simulink library "lib_Clutchless_HSC"  (R2017b)
settings: Solver=VariableStepAuto  StartTime=0.0  StopTime=10.0  RelTol=1e-3
undefined symbols (not defined in the file): cal, eng, Engine, ENGTRQ_MSMCH_Degraded_CP, ENGTRQ_MSMCH_ErrCritical_CP, ENGTRQ_MSMCH_LimpHome_CP, gb, mot, tloop
libraries: simulink x83, EC2_libraries x4, powerlib_meascontrol x2, lib_SystemDiag x1, dspsigops x1
(part 4 of 6)

== system lib_Clutchless_HSC/Clutchless_HSC/HSC/Powertrain Manager/Torque Distribution/Supervisory  Control  Logic/VehReady.Sport_Mode.EngTrqCalc ==
  APP : Inport
  EngSpeed : Inport  Port=2
  Shifter : Inport  Port=3
  DrvIntdAxleTrq : Inport  Port=4
  TransRatio : Inport  Port=5
  f : TriggerPort  TriggerType=function-call  VariantControl=Variant
      settings: CopyFcn=Stateflow.SLINSF.SimulinkMan.removeBlockPreDeleteFcn  PreDeleteFcn=Stateflow.SLINSF.SimulinkMan.unsafePredeleteFcn
  Constant : Constant  Value=0
  Constant1 : Constant  Value=0
  Divide2 : Product  Inputs=**
  Divide3 : Product  Inputs=***
  Engine Max Trq : Lookup_n-D  NumberOfTableDimensions=1  BreakpointsForDimension1="[600\t800\t1000\t1200\t1400\t1600\t1800\t2000\t2200\t2400\t2600\t2800\t3000\t3200\t3400\t3600\t3800\t4000\t4250\t4500\t4750\t5000\t5250\t5500\t5750\t6000\t6250\t6500]"  Table="[83.7900000000000\t136.760000000000\t140\t152.010000000000\t171.590000000000\t185.900000000000\t198.400000000000\t197.360000000000\t200.550000000000\t202.260000000000\t215.080000000000\t204.810000000000\t204.520000000000\t208.100000000000\t211.520000000000\t210.560000000000\t214.100000000000\t213.470000000000\t208.730000000000\t208.430000000000\t208.670000000000\t231.210000000000\t228.310000000000\t225.330000000000\t220.520000000000\t211.210000000000\t204.190000000000\t151.770000000000]"  ExtrapMethod=Clip  UseLastTableValue=on  InternalRulePriority=Speed  RndMeth=Simplest  InputSameDT=on
  Final Drive Ratio : Constant  Value=fd.plant.init.ratio
  Index Vector : MultiPortSwitch  DataPortOrder=Zero-based contiguous  Inputs=5  zeroidx=on
  MinMax : MinMax  Inputs=2
  Saturation : Saturate  UpperLimit=230  LowerLimit=-inf
  to% : Gain  Gain=1/100
  T : Outport
  wires:
  MinMax/1 -> [TrqCalc]
  DrvIntdAxleTrq/1 -> MinMax/2
  Divide3/1 -> MinMax/1
  Final Drive Ratio/1 -> Divide3/3
  TransRatio/1 -> Divide3/2
  Divide2/1 -> Divide3/1
  Saturation/1 -> Divide2/2
  Engine Max Trq/1 -> Saturation/1
  EngSpeed/1 -> Engine Max Trq/1  "RPM"
  to%/1 -> Divide2/1
  APP/1 -> to%/1
  Shifter/1 -> Index Vector/1
  Index Vector/1 -> T/1
  [TrqCalc] -> Index Vector/5  "N"
  Constant1/1 -> Index Vector/3  "P"
  Constant/1 -> Index Vector/2  "Between Ranges"
  [TrqCalc] -> Index Vector/6  "D"
  [TrqCalc] -> Index Vector/4  "R"

== system lib_Clutchless_HSC/Clutchless_HSC/HSC/Powertrain Manager/Torque Distribution/Supervisory  Control  Logic/VehReady.Sport_Mode.MotTrqCalc ==
  APP : Inport
  Shifter : Inport  Port=2
  MotSpeed : Inport  Port=3
  DrvIntdAxleTrq : Inport  Port=4
  TransRatio : Inport  Port=5
  f : TriggerPort  TriggerType=function-call  VariantControl=Variant
      settings: CopyFcn=Stateflow.SLINSF.SimulinkMan.removeBlockPreDeleteFcn  PreDeleteFcn=Stateflow.SLINSF.SimulinkMan.unsafePredeleteFcn
  % to 1 : Gain  Gain=1/100
  Constant : Constant  Value=0
  Constant1 : Constant  Value=0
  Differential Ratio : Constant  Value=fd.plant.init.ratio
  Divide1 : Product  Inputs=**
  Divide2 : Product  Inputs=***
  Index Vector : MultiPortSwitch  DataPortOrder=Zero-based contiguous  Inputs=5  zeroidx=on
  MinMax : MinMax  Inputs=2
  Peak trq max - Motoring : Lookup  InputValues=mot.plant.init.regen.trq_max.idx1_spd  Table=mot.plant.init.motor.trq_max.map  LookUpMeth=Interpolation-Use End Values  SaturateOnIntegerOverflow=on
  T : Outport
  wires:
  MinMax/1 -> [TrqCalc]
  Divide2/1 -> MinMax/2
  DrvIntdAxleTrq/1 -> MinMax/1
  Differential Ratio/1 -> Divide2/3
  TransRatio/1 -> Divide2/2
  Divide1/1 -> Divide2/1
  Peak trq max - Motoring/1 -> Divide1/1
  MotSpeed/1 -> Peak trq max - Motoring/1  "RPM"
  APP/1 -> % to 1/1
  [TrqCalc] -> Index Vector/5  "N"
  Constant1/1 -> Index Vector/3  "P"
  Constant/1 -> Index Vector/2  "Between Ranges"
  Index Vector/1 -> T/1
  [TrqCalc] -> Index Vector/6  "D"
  [TrqCalc] -> Index Vector/4  "R"
  Shifter/1 -> Index Vector/1
  % to 1/1 -> Divide1/2

== system lib_Clutchless_HSC/Clutchless_HSC/HSC/Powertrain Manager/Torque Distribution/SysPwrMd ==
  note: Disable Engine if HVIL on
  note: Switch added to test engine start
      | 04/13/2017 - Sebastian
  SysPwrMd : Inport
  EngRunAtv : Inport  Port=2
  EngOnReq : Inport  Port=3
  Fehler_Pilot : Inport  Port=4
  Constant1 : Constant  Value=3
  Constant2 : Constant
  Constant3 : Constant  Value=0
  EngOnReq_Cal : Constant  Value=0
  Saturation2 : Saturate  UpperLimit=2  LowerLimit=0
  Saturation3 : Saturate  UpperLimit=2  LowerLimit=0
  Switch{1..5} (5 alike) : Switch  Threshold=1
  Out1 : Outport
  wires:
  Switch2/1 -> Switch3/3
  Constant1/1 -> Switch1/3
  Constant2/1 -> Switch2/1
  EngRunAtv/1 -> Switch2/2, Switch1/2
  Saturation2/1 -> Switch1/1
  SysPwrMd/1 -> Saturation3/1, Saturation2/1
  Saturation3/1 -> Switch2/3
  EngOnReq/1 -> Switch4/3
  Switch1/1 -> Switch3/1
  Switch3/1 -> Switch5/3
  EngOnReq_Cal/1 -> Switch4/2, Switch4/1
  Switch4/1 -> Switch3/2
  Fehler_Pilot/1 -> Switch5/2
  Switch5/1 -> Out1/1
  Constant3/1 -> Switch5/1

== system lib_Clutchless_HSC/Clutchless_HSC/HSC/Powertrain Manager/Torque Distribution/eSystemStatusValidity ==
  In1 : Inport
  " Normal Operation" : simulink/Logic and Bit Operations/Compare To Constant  relop===  const=2  OutDataTypeStr=boolean
  Limited Operation : simulink/Logic and Bit Operations/Compare To Constant  relop===  const=1  OutDataTypeStr=boolean
  Logical Operator : Logic  Operator=OR  AllPortsSameDT=off  OutDataTypeStr=boolean
  Out1 : Outport
  wires:
  In1/1 -> " Normal Operation"/1, Limited Operation/1
  Limited Operation/1 -> Logical Operator/1
  " Normal Operation"/1 -> Logical Operator/2
  Logical Operator/1 -> Out1/1

== system lib_Clutchless_HSC/Clutchless_HSC/HSC/Powertrain Manager/Torque Distribution/iceSystemStatusValidity ==
  In1 : Inport
  " Normal Operation" : simulink/Logic and Bit Operations/Compare To Constant  relop===  const=2  OutDataTypeStr=boolean
  Limited Operation : simulink/Logic and Bit Operations/Compare To Constant  relop===  const=1  OutDataTypeStr=boolean
  Logical Operator : Logic  Operator=OR  AllPortsSameDT=off  OutDataTypeStr=boolean
  Out1 : Outport
  wires:
  Logical Operator/1 -> Out1/1
  " Normal Operation"/1 -> Logical Operator/2
  Limited Operation/1 -> Logical Operator/1
  In1/1 -> Limited Operation/1, " Normal Operation"/1

== system lib_Clutchless_HSC/Clutchless_HSC/HSC/Camaro Fault Detection/Component Diagnostic/Engine Component Diagnostic/Override  engTrqCmd ==
  note: Override Switch Subsystem
  note: This subsystem is used to override the model value of a signal to a constant value
  In1 : Inport
  Constant : Constant  Value=50
  Multiport Switch : MultiPortSwitch  DataPortOrder=Zero-based contiguous  Inputs=2  zeroidx=on
  Signal Override Switch 0 = Use Model 1 = Use Constant : Constant
  Out1 : Outport
  wires:
  Constant/1 -> Multiport Switch/3
  Multiport Switch/1 -> Out1/1
  In1/1 -> Multiport Switch/2
  Signal Override Switch 0 = Use Model 1 = Use Constant/1 -> Multiport Switch/1

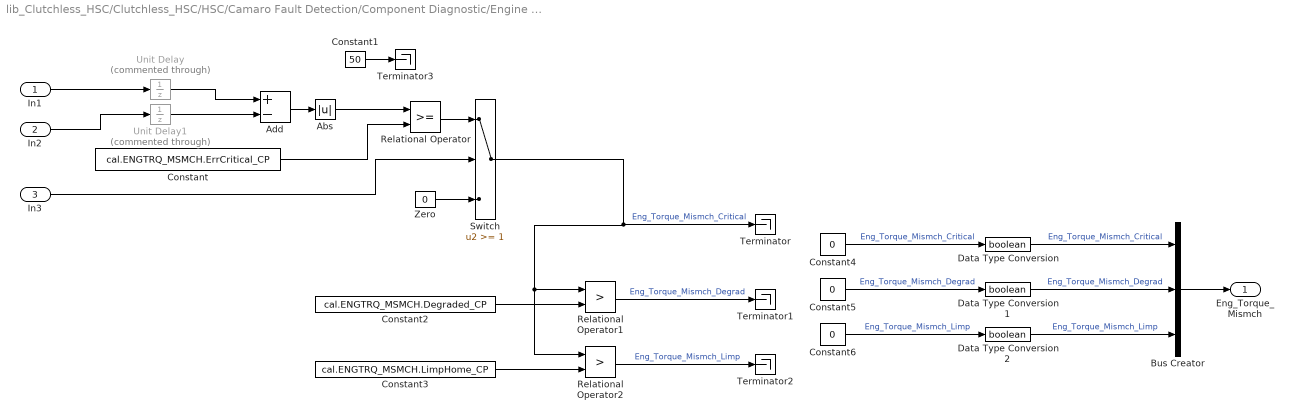
== system lib_Clutchless_HSC/Clutchless_HSC/HSC/Camaro Fault Detection/Component Diagnostic/Engine Component Diagnostic/TorqMismatch Detection ==
  In1 : Inport
  In2 : Inport  Port=2
  In3 : Inport  Port=3
  Abs : Abs
  Add : Sum  Inputs=+-
  Bus Creator : BusCreator  Inputs=3
  Constant : Constant  Value=cal.ENGTRQ_MSMCH.ErrCritical_CP
  Constant1 : Constant  Value=50
  Constant2 : Constant  Value=cal.ENGTRQ_MSMCH.Degraded_CP
  Constant3 : Constant  Value=cal.ENGTRQ_MSMCH.LimpHome_CP
  Constant4 : Constant  Value=0
  Constant5 : Constant  Value=0
  Constant6 : Constant  Value=0
  Data Type Conversion : DataTypeConversion  OutDataTypeStr=boolean
  Data Type Conversion1 : DataTypeConversion  OutDataTypeStr=boolean
  Data Type Conversion2 : DataTypeConversion  OutDataTypeStr=boolean
  Relational Operator : RelationalOperator  OutDataTypeStr=boolean  RndMeth=Nearest
  Relational Operator1 : RelationalOperator  Operator=>  OutDataTypeStr=boolean  RndMeth=Nearest
  Relational Operator2 : RelationalOperator  Operator=>  OutDataTypeStr=boolean  RndMeth=Nearest
  Switch : Switch  Threshold=1
  Terminator{,1..3} (4 alike) : Terminator
  Unit Delay : UnitDelay  Commented=through  SampleTime=-1
  Unit Delay1 : UnitDelay  Commented=through  SampleTime=-1
  "Zero " : Constant  Value=0
  Eng_Torque_Mismch : Outport
  wires:
  Data Type Conversion2/1 -> Bus Creator/3  "Eng_Torque_Mismch_Limp"
  Data Type Conversion1/1 -> Bus Creator/2  "Eng_Torque_Mismch_Degrad"
  Data Type Conversion/1 -> Bus Creator/1  "Eng_Torque_Mismch_Critical"
  Constant5/1 -> Data Type Conversion1/1  "Eng_Torque_Mismch_Degrad"
  Constant6/1 -> Data Type Conversion2/1  "Eng_Torque_Mismch_Limp"
  Constant4/1 -> Data Type Conversion/1  "Eng_Torque_Mismch_Critical"
  Abs/1 -> Relational Operator/1
  Unit Delay1/1 -> Add/2
  Bus Creator/1 -> Eng_Torque_Mismch/1
  Relational Operator2/1 -> Terminator2/1  "Eng_Torque_Mismch_Limp"
  Relational Operator1/1 -> Terminator1/1  "Eng_Torque_Mismch_Degrad"
  Constant3/1 -> Relational Operator2/2
  Constant2/1 -> Relational Operator1/2
  Switch/1 -> Terminator/1, Relational Operator1/1, Relational Operator2/1  "Eng_Torque_Mismch_Critical"
  Relational Operator/1 -> Switch/1
  Add/1 -> Abs/1
  Constant/1 -> Relational Operator/2
  Unit Delay/1 -> Add/1
  In3/1 -> Switch/2
  "Zero "/1 -> Switch/3
  In2/1 -> Unit Delay1/1
  In1/1 -> Unit Delay/1
  Constant1/1 -> Terminator3/1

== system lib_Clutchless_HSC/Clutchless_HSC/HSC/Camaro Fault Detection/Input Conversions/BMS_Conversions/Override  BMS_gdf 0_1 ==
  note: This subsystem is used to override the model value of a signal to a constant value
  note: Override Switch Subsystem
  In1 : Inport
  Multiport Switch : MultiPortSwitch  DataPortOrder=Zero-based contiguous  Inputs=2  zeroidx=on
  Override Value : Constant  Value=0  OutDataTypeStr=double
  Signal Override Switch 0 = Use Model 1 = Use Constant : Constant
  Out1 : Outport
  wires:
  Signal Override Switch 0 = Use Model 1 = Use Constant/1 -> Multiport Switch/1
  In1/1 -> Multiport Switch/2
  Multiport Switch/1 -> Out1/1
  Override Value/1 -> Multiport Switch/3

== system lib_Clutchless_HSC/Clutchless_HSC/HSC/Camaro Fault Detection/Input Conversions/BMS_Conversions/Override  closeContactorsCmd ==
  note: Override Switch Subsystem
  note: This subsystem is used to override the model value of a signal to a constant value
  In1 : Inport
  Multiport Switch : MultiPortSwitch  DataPortOrder=Zero-based contiguous  Inputs=2  zeroidx=on
  Override Value : Constant  Value=0  OutDataTypeStr=double
  Signal Override Switch 0 = Use Model 1 = Use Constant : Constant  Value=0
  Out1 : Outport
  wires:
  Override Value/1 -> Multiport Switch/3
  Multiport Switch/1 -> Out1/1
  In1/1 -> Multiport Switch/2
  Signal Override Switch 0 = Use Model 1 = Use Constant/1 -> Multiport Switch/1

== system lib_Clutchless_HSC/Clutchless_HSC/HSC/Camaro Fault Detection/Input Conversions/BMS_Conversions/Override  contactorsClsd ==
  note: Override Switch Subsystem
  note: This subsystem is used to override the model value of a signal to a constant value
  In1 : Inport
  Multiport Switch : MultiPortSwitch  DataPortOrder=Zero-based contiguous  Inputs=2  zeroidx=on
  Override Value : Constant  Value=0  OutDataTypeStr=double
  Signal Override Switch 0 = Use Model 1 = Use Constant : Constant  Value=0
  Out1 : Outport
  wires:
  Override Value/1 -> Multiport Switch/3
  Multiport Switch/1 -> Out1/1
  In1/1 -> Multiport Switch/2
  Signal Override Switch 0 = Use Model 1 = Use Constant/1 -> Multiport Switch/1

== system lib_Clutchless_HSC/Clutchless_HSC/HSC/Camaro Fault Detection/Input Conversions/BMS_Conversions/Override  essCur_A ==
  note: This subsystem is used to override the model value of a signal to a constant value
  note: Override Switch Subsystem
  In1 : Inport
  Multiport Switch : MultiPortSwitch  DataPortOrder=Zero-based contiguous  Inputs=2  zeroidx=on
  Override Value : Constant  Value=0  OutDataTypeStr=double
  Signal Override Switch 0 = Use Model 1 = Use Constant : Constant  Value=0
  Out1 : Outport
  wires:
  Signal Override Switch 0 = Use Model 1 = Use Constant/1 -> Multiport Switch/1
  In1/1 -> Multiport Switch/2
  Multiport Switch/1 -> Out1/1
  Override Value/1 -> Multiport Switch/3

== system lib_Clutchless_HSC/Clutchless_HSC/HSC/Camaro Fault Detection/Input Conversions/BMS_Conversions/Override  essSOC_0_1 ==
  note: Override Switch Subsystem
  note: This subsystem is used to override the model value of a signal to a constant value
  In1 : Inport
  Multiport Switch : MultiPortSwitch  DataPortOrder=Zero-based contiguous  Inputs=2  zeroidx=on
  Override Value : Constant  Value=0  OutDataTypeStr=double
  Signal Override Switch 0 = Use Model 1 = Use Constant : Constant  Value=0
  Out1 : Outport
  wires:
  Override Value/1 -> Multiport Switch/3
  Multiport Switch/1 -> Out1/1
  In1/1 -> Multiport Switch/2
  Signal Override Switch 0 = Use Model 1 = Use Constant/1 -> Multiport Switch/1

== system lib_Clutchless_HSC/Clutchless_HSC/HSC/Camaro Fault Detection/Input Conversions/BMS_Conversions/Override  essTemp_C ==
  note: Override Switch Subsystem
  note: This subsystem is used to override the model value of a signal to a constant value
  In1 : Inport
  Multiport Switch : MultiPortSwitch  DataPortOrder=Zero-based contiguous  Inputs=2  zeroidx=on
  Override Value : Constant  Value=0  OutDataTypeStr=double
  Signal Override Switch 0 = Use Model 1 = Use Constant : Constant
  Out1 : Outport
  wires:
  Override Value/1 -> Multiport Switch/3
  Multiport Switch/1 -> Out1/1
  In1/1 -> Multiport Switch/2
  Signal Override Switch 0 = Use Model 1 = Use Constant/1 -> Multiport Switch/1

== system lib_Clutchless_HSC/Clutchless_HSC/HSC/Camaro Fault Detection/Input Conversions/BMS_Conversions/Override  hvBattVolt_V ==
  note: Override Switch Subsystem
  note: This subsystem is used to override the model value of a signal to a constant value
  In1 : Inport
  Multiport Switch : MultiPortSwitch  DataPortOrder=Zero-based contiguous  Inputs=2  zeroidx=on
  Override Value : Constant  Value=0  OutDataTypeStr=double
  Signal Override Switch 0 = Use Model 1 = Use Constant : Constant  Value=0
  Out1 : Outport
  wires:
  Override Value/1 -> Multiport Switch/3
  Multiport Switch/1 -> Out1/1
  In1/1 -> Multiport Switch/2
  Signal Override Switch 0 = Use Model 1 = Use Constant/1 -> Multiport Switch/1

== system lib_Clutchless_HSC/Clutchless_HSC/HSC/Camaro Fault Detection/Input Conversions/BMS_Conversions/Override  hvBusVolt_V ==
  note: This subsystem is used to override the model value of a signal to a constant value
  note: Override Switch Subsystem
  In1 : Inport
  Multiport Switch : MultiPortSwitch  DataPortOrder=Zero-based contiguous  Inputs=2  zeroidx=on
  Override Value : Constant  Value=0  OutDataTypeStr=double
  Signal Override Switch 0 = Use Model 1 = Use Constant : Constant  Value=0
  Out1 : Outport
  wires:
  Signal Override Switch 0 = Use Model 1 = Use Constant/1 -> Multiport Switch/1
  In1/1 -> Multiport Switch/2
  Multiport Switch/1 -> Out1/1
  Override Value/1 -> Multiport Switch/3

== system lib_Clutchless_HSC/Clutchless_HSC/HSC/Camaro Fault Detection/Input Conversions/BMS_Conversions/Override  rollingAliveCnt [1_3] ==
  note: This subsystem is used to override the model value of a signal to a constant value
  note: Override Switch Subsystem
  In1 : Inport
  Multiport Switch : MultiPortSwitch  DataPortOrder=Zero-based contiguous  Inputs=2  zeroidx=on
  Override Value : Constant  Value=0  OutDataTypeStr=double
  Signal Override Switch 0 = Use Model 1 = Use Constant : Constant  Value=0
  Out1 : Outport
  wires:
  Signal Override Switch 0 = Use Model 1 = Use Constant/1 -> Multiport Switch/1
  In1/1 -> Multiport Switch/2
  Multiport Switch/1 -> Out1/1
  Override Value/1 -> Multiport Switch/3

== system lib_Clutchless_HSC/Clutchless_HSC/HSC/Camaro Fault Detection/Input Conversions/BMS_Conversions/Override Fehler_HS_offen ==
  note: Override Switch Subsystem
  note: This subsystem is used to override the model value of a signal to a constant value
  In1 : Inport
  Multiport Switch : MultiPortSwitch  DataPortOrder=Zero-based contiguous  Inputs=2  zeroidx=on
  Override Value : Constant  Value=0  OutDataTypeStr=double
  Signal Override Switch 0 = Use Model 1 = Use Constant : Constant
  Out1 : Outport
  wires:
  Override Value/1 -> Multiport Switch/3
  Multiport Switch/1 -> Out1/1
  In1/1 -> Multiport Switch/2
  Signal Override Switch 0 = Use Model 1 = Use Constant/1 -> Multiport Switch/1

== system lib_Clutchless_HSC/Clutchless_HSC/HSC/Camaro Fault Detection/Input Conversions/BMS_Conversions/Override Fehler_HS_verschweisst ==
  note: This subsystem is used to override the model value of a signal to a constant value
  note: Override Switch Subsystem
  In1 : Inport
  Multiport Switch : MultiPortSwitch  DataPortOrder=Zero-based contiguous  Inputs=2  zeroidx=on
  Override Value : Constant  Value=0  OutDataTypeStr=double
  Signal Override Switch 0 = Use Model 1 = Use Constant : Constant
  Out1 : Outport
  wires:
  Signal Override Switch 0 = Use Model 1 = Use Constant/1 -> Multiport Switch/1
  In1/1 -> Multiport Switch/2
  Multiport Switch/1 -> Out1/1
  Override Value/1 -> Multiport Switch/3

== system lib_Clutchless_HSC/Clutchless_HSC/HSC/Camaro Fault Detection/Input Conversions/DriverInput_Conversions/Override  KeyPos [0_3] ==
  note: This subsystem is used to override the model value of a signal to a constant value
  note: Override Switch Subsystem
  In1 : Inport
  Multiport Switch : MultiPortSwitch  DataPortOrder=Zero-based contiguous  Inputs=2  zeroidx=on
  Override Value : Constant  Value=0  OutDataTypeStr=double
  Signal Override Switch 0 = Use Model 1 = Use Constant : Constant  Value=0
  Out1 : Outport
  wires:
  Signal Override Switch 0 = Use Model 1 = Use Constant/1 -> Multiport Switch/1
  In1/1 -> Multiport Switch/2
  Multiport Switch/1 -> Out1/1
  Override Value/1 -> Multiport Switch/3

== system lib_Clutchless_HSC/Clutchless_HSC/HSC/Camaro Fault Detection/Input Conversions/DriverInput_Conversions/Override APP (%) ==
  note: This subsystem is used to override the model value of a signal to a constant value
  note: Override Switch Subsystem
  In1 : Inport
  Multiport Switch : MultiPortSwitch  DataPortOrder=Zero-based contiguous  Inputs=2  zeroidx=on
  Override Value : Constant  Value=0  OutDataTypeStr=double
  Signal Override Switch 0 = Use Model 1 = Use Constant : Constant  Value=0
  Out1 : Outport
  wires:
  Signal Override Switch 0 = Use Model 1 = Use Constant/1 -> Multiport Switch/1
  In1/1 -> Multiport Switch/2
  Multiport Switch/1 -> Out1/1
  Override Value/1 -> Multiport Switch/3

== system lib_Clutchless_HSC/Clutchless_HSC/HSC/Camaro Fault Detection/Input Conversions/DriverInput_Conversions/Override APP (%)1 ==
  note: Override Switch Subsystem
  note: This subsystem is used to override the model value of a signal to a constant value
  In1 : Inport
  Multiport Switch : MultiPortSwitch  DataPortOrder=Zero-based contiguous  Inputs=2  zeroidx=on
  Override Value : Constant  Value=0  OutDataTypeStr=double
  Signal Override Switch 0 = Use Model 1 = Use Constant : Constant  Value=0
  Out1 : Outport
  wires:
  Override Value/1 -> Multiport Switch/3
  Multiport Switch/1 -> Out1/1
  In1/1 -> Multiport Switch/2
  Signal Override Switch 0 = Use Model 1 = Use Constant/1 -> Multiport Switch/1

== system lib_Clutchless_HSC/Clutchless_HSC/HSC/Camaro Fault Detection/Input Conversions/DriverInput_Conversions/Override BPP (%) ==
  note: Override Switch Subsystem
  note: This subsystem is used to override the model value of a signal to a constant value
  In1 : Inport
  Multiport Switch : MultiPortSwitch  DataPortOrder=Zero-based contiguous  Inputs=2  zeroidx=on
  Override Value : Constant  Value=0  OutDataTypeStr=double
  Signal Override Switch 0 = Use Model 1 = Use Constant : Constant  Value=0
  Out1 : Outport
  wires:
  Override Value/1 -> Multiport Switch/3
  Multiport Switch/1 -> Out1/1
  In1/1 -> Multiport Switch/2
  Signal Override Switch 0 = Use Model 1 = Use Constant/1 -> Multiport Switch/1

== system lib_Clutchless_HSC/Clutchless_HSC/HSC/Camaro Fault Detection/Input Conversions/DriverInput_Conversions/Override PRNDL ==
  note: This subsystem is used to override the model value of a signal to a constant value
  note: Override Switch Subsystem
  In1 : Inport
  Multiport Switch : MultiPortSwitch  DataPortOrder=Zero-based contiguous  Inputs=2  zeroidx=on
  Override Value : Constant  Value=0  OutDataTypeStr=double
  Signal Override Switch 0 = Use Model 1 = Use Constant : Constant  Value=0
  Out1 : Outport
  wires:
  Signal Override Switch 0 = Use Model 1 = Use Constant/1 -> Multiport Switch/1
  In1/1 -> Multiport Switch/2
  Multiport Switch/1 -> Out1/1
  Override Value/1 -> Multiport Switch/3

== system lib_Clutchless_HSC/Clutchless_HSC/HSC/Camaro Fault Detection/Input Conversions/DriverInput_Conversions/Override Regen ==
  note: This subsystem is used to override the model value of a signal to a constant value
  note: Override Switch Subsystem
  In1 : Inport
  Multiport Switch : MultiPortSwitch  DataPortOrder=Zero-based contiguous  Inputs=2  zeroidx=on
  Override Value : Constant  Value=0  OutDataTypeStr=double
  Signal Override Switch 0 = Use Model 1 = Use Constant : Constant  Value=0
  Out1 : Outport
  wires:
  Signal Override Switch 0 = Use Model 1 = Use Constant/1 -> Multiport Switch/1
  In1/1 -> Multiport Switch/2
  Multiport Switch/1 -> Out1/1
  Override Value/1 -> Multiport Switch/3

== system lib_Clutchless_HSC/Clutchless_HSC/HSC/Camaro Fault Detection/Input Conversions/DriverInput_Conversions/Override V [mph] ==
  note: Override Switch Subsystem
  note: This subsystem is used to override the model value of a signal to a constant value
  In1 : Inport
  Multiport Switch : MultiPortSwitch  DataPortOrder=Zero-based contiguous  Inputs=2  zeroidx=on
  Override Value : Constant  Value=0  OutDataTypeStr=double
  Signal Override Switch 0 = Use Model 1 = Use Constant : Constant  Value=0
  Out1 : Outport
  wires:
  Override Value/1 -> Multiport Switch/3
  Multiport Switch/1 -> Out1/1
  In1/1 -> Multiport Switch/2
  Signal Override Switch 0 = Use Model 1 = Use Constant/1 -> Multiport Switch/1

== system lib_Clutchless_HSC/Clutchless_HSC/HSC/Camaro Fault Detection/Input Conversions/ECM_Conversions/Override  ECMTrqCmd_Nm ==
  note: Override Switch Subsystem
  note: This subsystem is used to override the model value of a signal to a constant value
  In1 : Inport
  Multiport Switch : MultiPortSwitch  DataPortOrder=Zero-based contiguous  Inputs=2  zeroidx=on
  Override Value : Constant  Value=0  OutDataTypeStr=double
  Signal Override Switch 0 = Use Model 1 = Use Constant : Constant  Value=0
  Out1 : Outport
  wires:
  Override Value/1 -> Multiport Switch/3
  Multiport Switch/1 -> Out1/1
  In1/1 -> Multiport Switch/2
  Signal Override Switch 0 = Use Model 1 = Use Constant/1 -> Multiport Switch/1

== system lib_Clutchless_HSC/Clutchless_HSC/HSC/Camaro Fault Detection/Input Conversions/ECM_Conversions/Override  ECMrollingAliveCnt ==
  note: This subsystem is used to override the model value of a signal to a constant value
  note: Override Switch Subsystem
  In1 : Inport
  Multiport Switch : MultiPortSwitch  DataPortOrder=Zero-based contiguous  Inputs=2  zeroidx=on
  Override Value : Constant  Value=0  OutDataTypeStr=double
  Signal Override Switch 0 = Use Model 1 = Use Constant : Constant  Value=0
  Out1 : Outport
  wires:
  Signal Override Switch 0 = Use Model 1 = Use Constant/1 -> Multiport Switch/1
  In1/1 -> Multiport Switch/2
  Multiport Switch/1 -> Out1/1
  Override Value/1 -> Multiport Switch/3

== system lib_Clutchless_HSC/Clutchless_HSC/HSC/Camaro Fault Detection/Input Conversions/ECM_Conversions/Override  EngActStdyStTorq_Nm ==
  note: This subsystem is used to override the model value of a signal to a constant value
  note: Override Switch Subsystem
  In1 : Inport
  Multiport Switch : MultiPortSwitch  DataPortOrder=Zero-based contiguous  Inputs=2  zeroidx=on
  Override Value : Constant  Value=0  OutDataTypeStr=double
  Signal Override Switch 0 = Use Model 1 = Use Constant : Constant  Value=0
  Out1 : Outport
  wires:
  Signal Override Switch 0 = Use Model 1 = Use Constant/1 -> Multiport Switch/1
  In1/1 -> Multiport Switch/2
  Multiport Switch/1 -> Out1/1
  Override Value/1 -> Multiport Switch/3

== system lib_Clutchless_HSC/Clutchless_HSC/HSC/Camaro Fault Detection/Input Conversions/ECM_Conversions/Override  EngRunAtv ==
  note: Override Switch Subsystem
  note: This subsystem is used to override the model value of a signal to a constant value
  In1 : Inport
  Multiport Switch : MultiPortSwitch  DataPortOrder=Zero-based contiguous  Inputs=2  zeroidx=on
  Override Value : Constant  Value=0  OutDataTypeStr=double
  Signal Override Switch 0 = Use Model 1 = Use Constant : Constant  Value=0
  Out1 : Outport
  wires:
  Override Value/1 -> Multiport Switch/3
  Multiport Switch/1 -> Out1/1
  In1/1 -> Multiport Switch/2
  Signal Override Switch 0 = Use Model 1 = Use Constant/1 -> Multiport Switch/1

== system lib_Clutchless_HSC/Clutchless_HSC/HSC/Camaro Fault Detection/Input Conversions/ECM_Conversions/Override  EngineSpeed_rpm ==
  note: Override Switch Subsystem
  note: This subsystem is used to override the model value of a signal to a constant value
  In1 : Inport
  Multiport Switch : MultiPortSwitch  DataPortOrder=Zero-based contiguous  Inputs=2  zeroidx=on
  Override Value : Constant  Value=0  OutDataTypeStr=double
  Signal Override Switch 0 = Use Model 1 = Use Constant : Constant  Value=0
  Out1 : Outport
  wires:
  Override Value/1 -> Multiport Switch/3
  Multiport Switch/1 -> Out1/1
  In1/1 -> Multiport Switch/2
  Signal Override Switch 0 = Use Model 1 = Use Constant/1 -> Multiport Switch/1

== system lib_Clutchless_HSC/Clutchless_HSC/HSC/Camaro Fault Detection/Input Conversions/ECM_Conversions/Override  Engine_Temp[DegC] ==
  note: This subsystem is used to override the model value of a signal to a constant value
  note: Override Switch Subsystem
  In1 : Inport
  Multiport Switch : MultiPortSwitch  DataPortOrder=Zero-based contiguous  Inputs=2  zeroidx=on
  Override Value : Constant  Value=0  OutDataTypeStr=double
  Signal Override Switch 0 = Use Model 1 = Use Constant : Constant  Value=0
  Out1 : Outport
  wires:
  Signal Override Switch 0 = Use Model 1 = Use Constant/1 -> Multiport Switch/1
  In1/1 -> Multiport Switch/2
  Multiport Switch/1 -> Out1/1
  Override Value/1 -> Multiport Switch/3

== system lib_Clutchless_HSC/Clutchless_HSC/HSC/Camaro Fault Detection/Input Conversions/TCM_Conversions/Override  LockupCmd ==
  note: Override Switch Subsystem
  note: This subsystem is used to override the model value of a signal to a constant value
  In1 : Inport
  Multiport Switch : MultiPortSwitch  DataPortOrder=Zero-based contiguous  Inputs=2  zeroidx=on
  Override Value : Constant  Value=0  OutDataTypeStr=double
  Signal Override Switch 0 = Use Model 1 = Use Constant : Constant  Value=0
  Out1 : Outport
  wires:
  Override Value/1 -> Multiport Switch/3
  Multiport Switch/1 -> Out1/1
  In1/1 -> Multiport Switch/2
  Signal Override Switch 0 = Use Model 1 = Use Constant/1 -> Multiport Switch/1

== system lib_Clutchless_HSC/Clutchless_HSC/HSC/Camaro Fault Detection/Input Conversions/TCM_Conversions/Override  LvrPosTrnsShft  ==
  note: Override Switch Subsystem
  note: This subsystem is used to override the model value of a signal to a constant value
  In1 : Inport
  Multiport Switch : MultiPortSwitch  DataPortOrder=Zero-based contiguous  Inputs=2  zeroidx=on
  Override Value : Constant  Value=0  OutDataTypeStr=double
  Signal Override Switch 0 = Use Model 1 = Use Constant : Constant  Value=0
  Out1 : Outport
  wires:
  Override Value/1 -> Multiport Switch/3
  Multiport Switch/1 -> Out1/1
  In1/1 -> Multiport Switch/2
  Signal Override Switch 0 = Use Model 1 = Use Constant/1 -> Multiport Switch/1

== system lib_Clutchless_HSC/Clutchless_HSC/HSC/Camaro Fault Detection/Input Conversions/TCM_Conversions/Override  TransEstGear ==
  note: Override Switch Subsystem
  note: This subsystem is used to override the model value of a signal to a constant value
  In1 : Inport
  Multiport Switch : MultiPortSwitch  DataPortOrder=Zero-based contiguous  Inputs=2  zeroidx=on
  Override Value : Constant  Value=0  OutDataTypeStr=double
  Signal Override Switch 0 = Use Model 1 = Use Constant : Constant  Value=0
  Out1 : Outport
  wires:
  Override Value/1 -> Multiport Switch/3
  Multiport Switch/1 -> Out1/1
  In1/1 -> Multiport Switch/2
  Signal Override Switch 0 = Use Model 1 = Use Constant/1 -> Multiport Switch/1

== system lib_Clutchless_HSC/Clutchless_HSC/HSC/Camaro Fault Detection/Input Conversions/TCM_Conversions/Override  rollingAliveCnt [123] ==
  note: Override Switch Subsystem
  note: This subsystem is used to override the model value of a signal to a constant value
  In1 : Inport
  Multiport Switch : MultiPortSwitch  DataPortOrder=Zero-based contiguous  Inputs=2  zeroidx=on
  Override Value : Constant  Value=0  OutDataTypeStr=double
  Signal Override Switch 0 = Use Model 1 = Use Constant : Constant  Value=0
  Out1 : Outport
  wires:
  Override Value/1 -> Multiport Switch/3
  Multiport Switch/1 -> Out1/1
  In1/1 -> Multiport Switch/2
  Signal Override Switch 0 = Use Model 1 = Use Constant/1 -> Multiport Switch/1

== system lib_Clutchless_HSC/Clutchless_HSC/HSC/Camaro Fault Detection/Input Conversions/TCM_Conversions/TCM_RollinAliveCounter ==
  Constant : Constant  Value=0
  Constant8 : Constant
  Rolling Alive Counter1 : Stateflow chart  TreatAsAtomicUnit=on
  Switch1 : Switch  Criteria=u2 > Threshold
  Out1 : Outport
  wires:
  Constant8/1 -> Switch1/1
  Rolling Alive Counter1/1(RollingAliveCnt) -> Switch1/3
  [TCM_CAN_fault] -> Switch1/2
  Switch1/1 -> Out1/1  "TCMRollingAliveCnt [0 1 2 3]"
  Constant/1 -> [TCM_CAN_fault]

== system lib_Clutchless_HSC/Clutchless_HSC/HSC/Camaro Fault Detection/Signal Diagnostic/Driver Signal Diagnostic/APP_Crosscheck ==
  In1 : Inport
  In2 : Inport  Port=2
  Abs : Abs
  Compare To Constant : simulink/Logic and Bit Operations/Compare To Constant  relop=<=  const=0.5  OutDataTypeStr=boolean
  Sum : Sum  Inputs=+-
  Out1 : Outport
  wires:
  Compare To Constant/1 -> Out1/1  "Drv_APP_Agree"
  In2/1 -> Sum/2
  In1/1 -> Sum/1
  Abs/1 -> Compare To Constant/1
  Sum/1 -> Abs/1

== system lib_Clutchless_HSC/Clutchless_HSC/HSC/Camaro Fault Detection/Signal Diagnostic/Driver Signal Diagnostic/BrakeFailureDetection ==
  BPP : Inport
  VehSpeed : Inport  Port=2
  Trigger : TriggerPort  VariantControl=Variant  PortDimensions=1
  Chart : Stateflow chart  Commented=on  TreatAsAtomicUnit=on
  Compare To Constant : simulink/Logic and Bit Operations/Compare To Constant  relop=>  const=0  OutDataTypeStr=boolean
  Compare To Constant1 : simulink/Logic and Bit Operations/Compare To Constant  relop=>  const=0.5  OutDataTypeStr=boolean
  Detect Change : simulink/Logic and Bit Operations/Detect Change  vinit=0  InputProcessing=Inherited  OutDataTypeStr=boolean
  Detect Increase : simulink/Logic and Bit Operations/Detect Increase  vinit=0.0  InputProcessing=Inherited  OutDataTypeStr=boolean
  Logical Operator : Logic  Operator=NOT  AllPortsSameDT=off  OutDataTypeStr=boolean
  Logical Operator1 : Logic  AllPortsSameDT=off  OutDataTypeStr=boolean
  Logical Operator2 : Logic  Operator=OR  AllPortsSameDT=off  OutDataTypeStr=boolean
  Logical Operator3 : Logic  AllPortsSameDT=off  OutDataTypeStr=boolean
  Unit Delay : UnitDelay  SampleTime=-1
  Unit Delay1 : UnitDelay  SampleTime=-1
  DecelFail : Outport
  wires:
  Logical Operator3/1 -> DecelFail/1
  Logical Operator2/1 -> Logical Operator3/2
  Unit Delay1/1 -> Compare To Constant1/1
  Unit Delay/1 -> Compare To Constant/1
  Logical Operator/1 -> Logical Operator2/2  "Unchange"
  Detect Increase/1 -> Logical Operator2/1  "Increase"
  Logical Operator1/1 -> Logical Operator3/1
  BPP/1 -> Unit Delay/1
  Compare To Constant1/1 -> Logical Operator1/2
  Compare To Constant/1 -> Logical Operator1/1
  Detect Change/1 -> Logical Operator/1
  VehSpeed/1 -> Detect Increase/1, Detect Change/1, Unit Delay1/1

== system lib_Clutchless_HSC/Clutchless_HSC/HSC/Camaro Fault Detection/Signal Diagnostic/Driver Signal Diagnostic/Latch ==
  In1 : Inport
  In2 : Inport  Port=2
  Memory : Memory
  NOT : Logic  Operator=NOT  OutDataTypeStr=boolean
  OR : Logic  OutDataTypeStr=boolean
  OR1 : Logic  Operator=OR  OutDataTypeStr=boolean
  Drv_APP_Agree : Outport
  wires:
  In2/1 -> NOT/1
  Memory/1 -> OR/2
  NOT/1 -> OR/1
  OR1/1 -> Memory/1, Drv_APP_Agree/1
  OR/1 -> OR1/2
  In1/1 -> OR1/1

== system lib_Clutchless_HSC/Clutchless_HSC/HSC/Camaro Fault Detection/Signal Diagnostic/Driver Signal Diagnostic/Latch1 ==
  In1 : Inport
  In2 : Inport  Port=2
  Memory : Memory
  NOT : Logic  Operator=NOT  OutDataTypeStr=boolean
  OR : Logic  OutDataTypeStr=boolean
  OR1 : Logic  Operator=OR  OutDataTypeStr=boolean
  Out1 : Outport
  wires:
  In1/1 -> OR1/1
  OR/1 -> OR1/2
  OR1/1 -> Out1/1, Memory/1
  NOT/1 -> OR/1
  Memory/1 -> OR/2
  In2/1 -> NOT/1

== system lib_Clutchless_HSC/Clutchless_HSC/HSC/Camaro Fault Detection/Signal Diagnostic/ESS Signal Diagnostic/Contactors status check ==
  note: Note: Contactors don't close when commanded
  In1 : Inport
  In2 : Inport  Port=2
  In3 : Inport  Port=3
  " " : simulink/Logic and Bit Operations/Compare To Constant  relop=>  const=0.5  OutDataTypeStr=boolean
  Abs : Abs
  Logical Operator : Logic  Operator=OR  AllPortsSameDT=off  OutDataTypeStr=boolean
  Sum : Sum  Inputs=+-
  Out1 : Outport
  wires:
  In1/1 -> Sum/1
  Logical Operator/1 -> Out1/1  "BMS_contactorsFailed_Detected"
  Sum/1 -> Abs/1
  Abs/1 -> " "/1
  In2/1 -> Sum/2
  In3/1 -> Logical Operator/2
  " "/1 -> Logical Operator/1  "BMS_contactorsFailed_SigValid"

== system lib_Clutchless_HSC/Clutchless_HSC/HSC/Camaro Fault Detection/Signal Diagnostic/ESS Signal Diagnostic/ESS SOC Validity Check ==
  In1 : Inport
  Constant1 : Constant
  essSOCValidity_Check : Subsystem
  essSOC_0_1Range : Stateflow chart  TreatAsAtomicUnit=on
  Out1 : Outport
  Out2 : Outport  Port=2
  wires:
  essSOC_0_1Range/1(essSOCRange) -> essSOCValidity_Check/1(In1), Out2/1
  Constant1/1 -> essSOC_0_1Range/1(clearFaults)
  In1/1 -> essSOC_0_1Range/2(signalValue)
  essSOCValidity_Check/1(Out1) -> Out1/1  "BMS_essSOC_0_1_SigValid"

== system lib_Clutchless_HSC/Clutchless_HSC/HSC/Camaro Fault Detection/Signal Diagnostic/ESS Signal Diagnostic/ESS Temp Validity Check ==
  In1 : Inport
  Constant : Constant
  essTsignalRange : Stateflow chart  TreatAsAtomicUnit=on
  essTsignalValidity_Check : Subsystem
  Out1 : Outport
  Out2 : Outport  Port=2
  wires:
  In1/1 -> essTsignalRange/2(signalValue)
  essTsignalRange/1(essTempRange) -> essTsignalValidity_Check/1(In1), Out2/1  "essTempRange[0_4]"
  essTsignalValidity_Check/1(Out1) -> Out1/1  "BMS_essTemp_[degC]_SigValid"
  Constant/1 -> essTsignalRange/1(clearFaults)

== system lib_Clutchless_HSC/Clutchless_HSC/HSC/Camaro Fault Detection/Signal Diagnostic/ESS Signal Diagnostic/Max charging voltage fault detect ==
  note: Note: When the ESS receives the energy from grid or regenerative braking,
      | the charging voltage to the inverter can not be bigger than 419V, otherwise the MCU will set to fault
  In1 : Inport
  " " : simulink/Logic and Bit Operations/Compare To Constant  relop=>  const=419  OutDataTypeStr=boolean
  Abs : Abs
  Compare To Zero : simulink/Logic and Bit Operations/Compare To Zero  relop=<  OutDataTypeStr=boolean
  Logical Operator : Logic  AllPortsSameDT=off  OutDataTypeStr=boolean
  Out1 : Outport
  wires:
  Abs/1 -> " "/1
  Logical Operator/1 -> Out1/1
  " "/1 -> Logical Operator/1
  In1/1 -> Compare To Zero/1, Abs/1
  Compare To Zero/1 -> Logical Operator/2

== system lib_Clutchless_HSC/Clutchless_HSC/HSC/Camaro Fault Detection/Signal Diagnostic/ESS Signal Diagnostic/Rolling Alive Counter Detection ==
  In1 : Inport
  Chart : Stateflow chart  TreatAsAtomicUnit=on
  Constant : Constant  Value=0.01
  Constant1 : Constant  Value=0.01
  Detect Change : simulink/Logic and Bit Operations/Detect Change  vinit=1  InputProcessing=Inherited  OutDataTypeStr=boolean
  Out1 : Outport
  wires:
  Constant1/1 -> Chart/3(tloop)
  In1/1 -> Detect Change/1
  Detect Change/1 -> Chart/1(PulseDetect)
  Chart/1(flag) -> Out1/1
  Constant/1 -> Chart/2(CycleTime)

== system lib_Clutchless_HSC/Clutchless_HSC/HSC/Camaro Fault Detection/Signal Diagnostic/ESS Signal Diagnostic/Validity Check ==
  In1 : Inport
  " Normal Operation" : simulink/Logic and Bit Operations/Compare To Constant  relop===  const=1  OutDataTypeStr=boolean
  Below Normal Operation : simulink/Logic and Bit Operations/Compare To Constant  relop===  const=0  OutDataTypeStr=boolean
  Logical Operator : Logic  Operator=OR  AllPortsSameDT=off  OutDataTypeStr=boolean
  Out1 : Outport
  wires:
  In1/1 -> Below Normal Operation/1, " Normal Operation"/1
  Below Normal Operation/1 -> Logical Operator/1
  " Normal Operation"/1 -> Logical Operator/2
  Logical Operator/1 -> Out1/1  "BMSgdf_SigValid"

== system lib_Clutchless_HSC/Clutchless_HSC/HSC/Camaro Fault Detection/Signal Diagnostic/Engine Signal Diagnostic/EngTempValidity_Check ==
  In1 : Inport
  Above Normal Operation : simulink/Logic and Bit Operations/Compare To Constant  relop===  const=3  OutDataTypeStr=boolean
  Logical Operator1 : Logic  Operator=NOT  AllPortsSameDT=off  OutDataTypeStr=boolean
  Out1 : Outport
  wires:
  Logical Operator1/1 -> Out1/1
  Above Normal Operation/1 -> Logical Operator1/1
  In1/1 -> Above Normal Operation/1

== system lib_Clutchless_HSC/Clutchless_HSC/HSC/Camaro Fault Detection/Signal Diagnostic/Engine Signal Diagnostic/Rolling Alive Counter Detection1 ==
  In1 : Inport
  Chart : Stateflow chart  TreatAsAtomicUnit=on
  Constant : Constant  Value=0.01
  Detect Change : simulink/Logic and Bit Operations/Detect Change  vinit=1  InputProcessing=Inherited  OutDataTypeStr=boolean
  Out1 : Outport
  wires:
  Constant/1 -> Chart/2(CycleTime)
  Chart/1(flag) -> Out1/1
  Detect Change/1 -> Chart/1(PulseDetect)
  In1/1 -> Detect Change/1

== system lib_Clutchless_HSC/Clutchless_HSC/HSC/Camaro Fault Detection/Signal Diagnostic/Transmission Signal Diagnostic/Rolling Alive Counter Detection ==
  In1 : Inport
  Chart : Stateflow chart  TreatAsAtomicUnit=on
  Constant : Constant  Value=0.01
  Detect Change : simulink/Logic and Bit Operations/Detect Change  vinit=1  InputProcessing=Inherited  OutDataTypeStr=boolean
  Out1 : Outport
  wires:
  Constant/1 -> Chart/2(CycleTime)
  Chart/1(flag) -> Out1/1
  Detect Change/1 -> Chart/1(PulseDetect)
  In1/1 -> Detect Change/1

== system lib_Clutchless_HSC/Clutchless_HSC/HSC/Camaro Fault Detection/Signal Diagnostic/Transmission Signal Diagnostic/Vehicle Direction Fault Detection ==
  LvrPosTrnsShft : Inport
  Speed : Inport  Port=2
  Compare To Constant : simulink/Logic and Bit Operations/Compare To Constant  relop===  const=4  OutDataTypeStr=boolean
  Compare To Constant1 : simulink/Logic and Bit Operations/Compare To Constant  relop=<  const=0  OutDataTypeStr=boolean
  Compare To Constant2 : simulink/Logic and Bit Operations/Compare To Constant  relop===  const=2  OutDataTypeStr=boolean
  Compare To Constant3 : simulink/Logic and Bit Operations/Compare To Constant  relop=>  const=0  OutDataTypeStr=boolean
  Logical Operator : Logic  AllPortsSameDT=off  OutDataTypeStr=boolean
  Logical Operator1 : Logic  AllPortsSameDT=off  OutDataTypeStr=boolean
  Logical Operator2 : Logic  Operator=OR  AllPortsSameDT=off  OutDataTypeStr=boolean
  Out1 : Outport
  wires:
  Logical Operator2/1 -> Out1/1
  Logical Operator/1 -> Logical Operator2/2
  Logical Operator1/1 -> Logical Operator2/1
  Compare To Constant3/1 -> Logical Operator1/2
  Compare To Constant2/1 -> Logical Operator1/1
  Compare To Constant/1 -> Logical Operator/1
  Compare To Constant1/1 -> Logical Operator/2
  Speed/1 -> Compare To Constant1/1, Compare To Constant3/1
  LvrPosTrnsShft/1 -> Compare To Constant/1, Compare To Constant2/1

== system lib_Clutchless_HSC/Clutchless_HSC/HSC/Driver_Requests/APP_BPP to DrvIntndAxlTrq2/Post Driver Intnded Axle Torque/Brake Command ==
  APP : Inport
  BPP : Inport  Port=2
  VehicleSpeed : Inport  Port=3
  1-D Lookup Table : Lookup_n-D  NumberOfTableDimensions=1  BreakpointsForDimension1=cal.Regen.BrakeAxleTrq.idx1_BrkPdlPos  Table=cal.Regen.BrakeAxleTrq.map  InternalRulePriority=Speed  RndMeth=Simplest  InputSameDT=on
  Compare To Constant : simulink/Logic and Bit Operations/Compare To Constant  relop=>=  const=cal.Regen.EnableSpeed  OutDataTypeStr=boolean
  Compare To Constant4 : simulink/Logic and Bit Operations/Compare To Constant  relop=<=  const=cal.Regen.EnableAPP  OutDataTypeStr=boolean
  Compare To Constant5 : simulink/Logic and Bit Operations/Compare To Constant  relop=>=  const=cal.Regen.DisableAPP  OutDataTypeStr=boolean
  Constant5 : Constant  Value=0
  Latch : Subsystem
  RegenCal : Gain  Gain=1.3
  Switch : Switch  Criteria=u2 > Threshold  Threshold=1
  Terminator : Terminator
  BrkAxlTrq : Outport
  wires:
  VehicleSpeed/1 -> Compare To Constant/1
  1-D Lookup Table/1 -> RegenCal/1
  Switch/1 -> BrkAxlTrq/1
  APP/1 -> Compare To Constant5/1, Compare To Constant4/1
  BPP/1 -> 1-D Lookup Table/1
  Compare To Constant/1 -> Switch/2
  Constant5/1 -> Switch/3
  Compare To Constant5/1 -> Latch/2(Reset)
  Compare To Constant4/1 -> Latch/1(Input)
  Latch/1(Out1) -> Terminator/1
  RegenCal/1 -> Switch/1

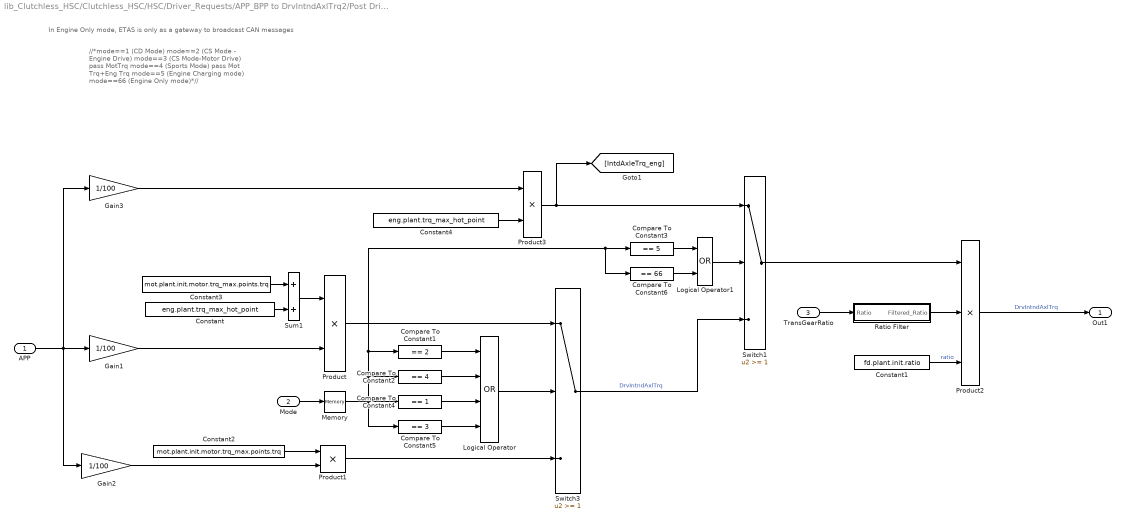
== system lib_Clutchless_HSC/Clutchless_HSC/HSC/Driver_Requests/APP_BPP to DrvIntndAxlTrq2/Post Driver Intnded Axle Torque/Driver Intended Axle Torque ==
  note: In Engine Only mode, ETAS is only as a gateway to broadcast CAN messages
  note: //*mode==1 (CD Mode)
      | mode==2 (CS Mode - Engine Drive)
      | mode==3 (CS Mode-Motor Drive) pass MotTrq
      | mode==4 (Sports Mode) pass Mot Trq+Eng Trq
      | mode==5 (Engine Charging mode)
      | mode==66 (Engine Only mode)*//
  APP : Inport
  Mode : Inport  Port=2
  TransGearRatio : Inport  Port=3
  Compare To Constant1 : simulink/Logic and Bit Operations/Compare To Constant  relop===  const=2  OutDataTypeStr=boolean
  Compare To Constant2 : simulink/Logic and Bit Operations/Compare To Constant  relop===  const=4  OutDataTypeStr=boolean
  Compare To Constant3 : simulink/Logic and Bit Operations/Compare To Constant  relop===  const=5  OutDataTypeStr=boolean
  Compare To Constant4 : simulink/Logic and Bit Operations/Compare To Constant  relop===  const=1  OutDataTypeStr=boolean
  Compare To Constant5 : simulink/Logic and Bit Operations/Compare To Constant  relop===  const=3  OutDataTypeStr=boolean
  Compare To Constant6 : simulink/Logic and Bit Operations/Compare To Constant  relop===  const=66  OutDataTypeStr=boolean
  Constant : Constant  Value=eng.plant.trq_max_hot_point  VectorParams1D=off
  Constant1 : Constant  Value=fd.plant.init.ratio
  Constant2 : Constant  Value=mot.plant.init.motor.trq_max.points.trq  VectorParams1D=off
  Constant3 : Constant  Value=mot.plant.init.motor.trq_max.points.trq  VectorParams1D=off
  Constant4 : Constant  Value=eng.plant.trq_max_hot_point  VectorParams1D=off
  Gain1 : Gain  Gain=1/100
  Gain2 : Gain  Gain=1/100
  Gain3 : Gain  Gain=1/100
  Logical Operator : Logic  Operator=OR  Inputs=4  AllPortsSameDT=off  OutDataTypeStr=boolean
  Logical Operator1 : Logic  Operator=OR  AllPortsSameDT=off  OutDataTypeStr=boolean
  Memory : Memory
  Product : Product  RndMeth=Zero
  Product1 : Product  RndMeth=Zero
  Product2 : Product  Inputs=3  RndMeth=Zero
  Product3 : Product  RndMeth=Zero
  Ratio Filter : Subsystem
  Sum1 : Sum
  Switch1 : Switch  Threshold=1
  Switch3 : Switch  Threshold=1
  Out1 : Outport
  wires:
  Constant2/1 -> Product1/1
  Ratio Filter/1(Filtered_Ratio) -> Product2/2
  Gain2/1 -> Product1/2
  Product/1 -> Switch3/1
  Mode/1 -> Memory/1
  Constant1/1 -> Product2/3  "ratio"
  Product1/1 -> Switch3/3
  TransGearRatio/1 -> Ratio Filter/1(Ratio)
  Product2/1 -> Out1/1  "DrvIntndAxlTrq"
  Gain1/1 -> Product/2
  Constant3/1 -> Sum1/1
  Compare To Constant1/1 -> Logical Operator/1
  Sum1/1 -> Product/1
  Compare To Constant2/1 -> Logical Operator/2
  Constant/1 -> Sum1/2
  Switch3/1 -> Switch1/3  "DrvIntndAxlTrq"
  Logical Operator/1 -> Switch3/2
  Product3/1 -> [IntdAxleTrq_eng], Switch1/1
  Switch1/1 -> Product2/1
  Compare To Constant3/1 -> Logical Operator1/1
  Memory/1 -> Compare To Constant2/1, Compare To Constant3/1, Compare To Constant6/1, Compare To Constant1/1, Compare To Constant4/1, Compare To Constant5/1
  APP/1 -> Gain2/1, Gain3/1, Gain1/1
  Constant4/1 -> Product3/2
  Gain3/1 -> Product3/1
  Logical Operator1/1 -> Switch1/2
  Compare To Constant6/1 -> Logical Operator1/2
  Compare To Constant4/1 -> Logical Operator/3
  Compare To Constant5/1 -> Logical Operator/4

== system lib_Clutchless_HSC/Clutchless_HSC/HSC/Powertrain Manager/HV Manager1/BMS_Manager/Fault Latch ==
  IsoFault : Inport
  Off Delay : powerlib_meascontrol/Logic/On Delay  DelayType=Off delay  delay=3  ic=0  Ts=0
      settings: SourceProductName=Simscape Power Systems
  IsoFaultLatched : Outport
  wires:
  IsoFault/1 -> Off Delay/1
  Off Delay/1 -> IsoFaultLatched/1

== system lib_Clutchless_HSC/Clutchless_HSC/HSC/Powertrain Manager/HV Manager1/BMS_Manager/ISO_Hybrid_01_Req ==
  In1 : Inport
  Bus Creator : BusCreator  Inputs=9
  ISO_Hybrid_01_Req_Data_byte_0 : Constant  Value=3
  ISO_Hybrid_01_Req_Data_byte_1 : Constant  Value=34
  ISO_Hybrid_01_Req_Data_byte_2 : Constant  Value=30
  ISO_Hybrid_01_Req_Data_byte_3 : Constant  Value=25
  ISO_Hybrid_01_Req_Data_byte_{4..7} (4 alike) : Constant  Value=0
  ISO_Hybrid_01_Req_Data_byte_8 : Constant  Value=23
  ISO_Request : DiscretePulseGenerator  PulseType=Time based  Period=0.5  PulseWidth=50  SampleTime=-1
  Switch{,1..8} (9 alike) : Switch  Criteria=u2 > Threshold
  Out1 : Outport
  wires:
  Bus Creator/1 -> Out1/1  "ISO_Hybrid_01_Req"
  Switch6/1 -> Bus Creator/6  "ISO_Hybrid_01_Req_Data_byte_5"
  ISO_Hybrid_01_Req_Data_byte_8/1 -> Switch/3
  Switch5/1 -> Bus Creator/5  "ISO_Hybrid_01_Req_Data_byte_4"
  Switch3/1 -> Bus Creator/3  "ISO_Hybrid_01_Req_Data_byte_2"
  ISO_Hybrid_01_Req_Data_byte_3/1 -> Switch/1
  Switch1/1 -> Bus Creator/1  "ISO_Hybrid_01_Req_Data_byte_0"
  Switch7/1 -> Bus Creator/7  "ISO_Hybrid_01_Req_Data_byte_6"
  Switch2/1 -> Bus Creator/2  "ISO_Hybrid_01_Req_Data_byte_1"
  Switch8/1 -> Bus Creator/8  "ISO_Hybrid_01_Req_Data_byte_7"
  Switch4/1 -> Bus Creator/4  "ISO_Hybrid_01_Req_Data_byte_3"
  ISO_Hybrid_01_Req_Data_byte_0/1 -> Switch1/1
  In1/1 -> Switch2/2, Switch3/3, Switch4/3, Switch5/3, Switch6/3, Switch7/2, Switch7/3, Switch8/2, Bus Creator/9, Switch8/3, Switch6/2, Switch5/2, Switch4/2, Switch3/2, Switch2/3, Switch1/3, Switch1/2
  ISO_Hybrid_01_Req_Data_byte_1/1 -> Switch2/1
  ISO_Hybrid_01_Req_Data_byte_2/1 -> Switch3/1
  Switch/1 -> Switch4/1  "ISO_Hybrid_01_Req_Data_byte_3"
  ISO_Hybrid_01_Req_Data_byte_4/1 -> Switch5/1
  ISO_Hybrid_01_Req_Data_byte_5/1 -> Switch6/1
  ISO_Hybrid_01_Req_Data_byte_6/1 -> Switch7/1
  ISO_Hybrid_01_Req_Data_byte_7/1 -> Switch8/1
  ISO_Request/1 -> Switch/2  "<ISO_Hybrid_01_Req_Data_byte_3>"

== system lib_Clutchless_HSC/Clutchless_HSC/HSC/Powertrain Manager/HV Manager1/BMS_Manager/Isolation Fault Calculation ==
  note: This block  allows to know which HV main
      | is having issues. HV POS 25, HV NEG 23.
  Sensors1 : Inport
  Bus Selector5 : BusSelector  OutputSignals=from_CAN.fromEBCAN.from_BMSAntrieb.ISO_Hybrid_01_Resp_Data.ISO_Hybrid_01_Resp_Data_byte_3,from_CAN.fromEBCAN.from_BMSAntrieb.ISO_Hybrid_01_Resp_Data.ISO_Hybrid_01_Resp_Data_byte_4,from_CAN.fromEBCAN.from_BMSAntrieb.ISO_Hybrid_01_Resp_Data.ISO_Hybrid_01_Resp_Data_byte_5
  Compare To Constant : simulink/Logic and Bit Operations/Compare To Constant  relop===  const=23  OutDataTypeStr=boolean
  Compare To Constant1 : simulink/Logic and Bit Operations/Compare To Constant  relop===  const=25  OutDataTypeStr=boolean
  HVnegativeISO : Constant  Value=0
  HVpositiveISO : Constant
  Logical Operator : Logic  Operator=OR  AllPortsSameDT=off  OutDataTypeStr=boolean
  POS or NEG HV MAIN : Switch  Criteria=u2 > Threshold  Threshold=24
  Resistance_Measurement : Subsystem
  Terminator8 : Terminator
  IsoFault : Outport
  wires:
  Resistance_Measurement/1(IsoFault) -> IsoFault/1
  POS or NEG HV MAIN/1 -> Terminator8/1
  Bus Selector5/2 -> Resistance_Measurement/1(In1)  "<ISO_Hybrid_01_Resp_Data_byte_4>"
  Bus Selector5/3 -> Resistance_Measurement/2(In2)  "<ISO_Hybrid_01_Resp_Data_byte_5>"
  Sensors1/1 -> Bus Selector5/1
  HVpositiveISO/1 -> POS or NEG HV MAIN/1
  Bus Selector5/1 -> POS or NEG HV MAIN/2, Compare To Constant1/1, Compare To Constant/1  "<ISO_Hybrid_01_Resp_Data_byte_3>"
  HVnegativeISO/1 -> POS or NEG HV MAIN/3
  Compare To Constant1/1 -> Logical Operator/1
  Compare To Constant/1 -> Logical Operator/2
  Logical Operator/1 -> Resistance_Measurement/Enable
